simulink model "Windowlifts_2017b"  (R2017b)
settings: Solver=FixedStepDiscrete  StartTime=0.0  StopTime=inf  FixedStep=0.0001  RelTol=1e-3
model workspace (MAT data in the model file):
  BCMU_permission = Simulink.Parameter
  BCMU_permission.Value = 1
  BCMU_permission.DataType = 'boolean'
  BCMU_permission.Min = 0
  BCMU_permission.Max = 1
  BCMU_permission.Dimensions = [1 1]
  driver_win_dn = Simulink.Parameter
  driver_win_dn.Value = 0
  driver_win_dn.DataType = 'boolean'
  driver_win_dn.Dimensions = [1 1]
  driver_win_up = Simulink.Parameter
  driver_win_up.Value = 0
  driver_win_up.DataType = 'boolean'
  driver_win_up.Dimensions = [1 1]
  mir_heater = Simulink.Parameter
  mir_heater.Value = 0
  mir_heater.Description = 'Rearview mirror heater switch request'
  mir_heater.DataType = 'boolean'
  mir_heater.Dimensions = [1 1]
  pass_win_dn = Simulink.Parameter
  pass_win_dn.Value = 0
  pass_win_dn.DataType = 'boolean'
  pass_win_dn.Dimensions = [1 1]
  pass_win_up = Simulink.Parameter
  pass_win_up.Value = 0
  pass_win_up.DataType = 'boolean'
  pass_win_up.Dimensions = [1 1]
  var_0 = Simulink.Parameter
  var_0.DataType = 'auto'
  var_0.Dimensions = [0 0]
libraries: simulink x2
settings Model: Creator=macbook  LastModifiedBy=junkie

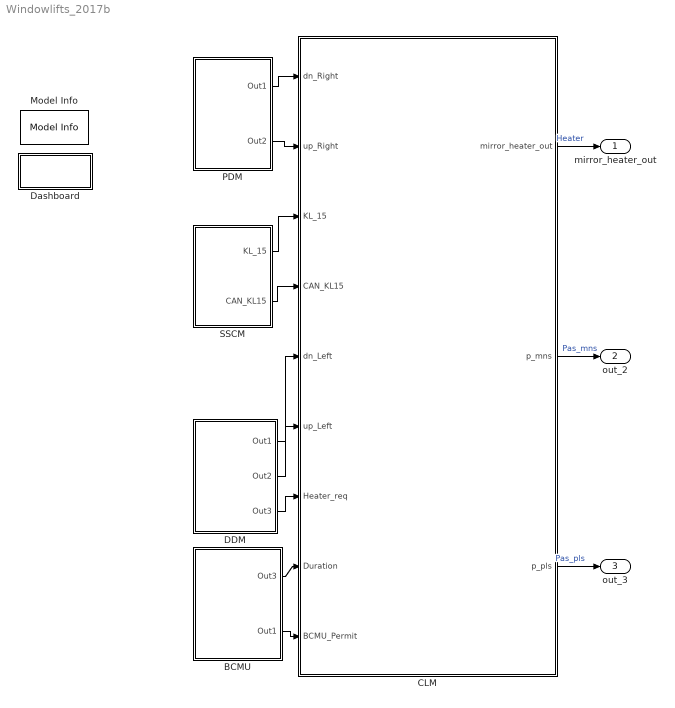
== system Windowlifts_2017b ==
  BCMU : Subsystem
  CLM : Subsystem
  DDM : Subsystem
  Dashboard : Subsystem  mask{Parameter2=<empty>}
      mask TypeOptions Parameter2: <empty>
  Model Info : simulink/Model-Wide Utilities/Model Info  Frame=on  DisplayStringWithTags=Model Info  HorizontalTextAlignment=Center  LeftAlignmentValue=0.5
  PDM : Subsystem
  SSCM : Subsystem
  mirror_heater_out : Outport
  out_2 : Outport  Port=2
  out_3 : Outport  Port=3
  wires:
  SSCM/1(KL_15) -> CLM/3(KL_15)
  SSCM/2(CAN_KL15) -> CLM/4(CAN_KL15)
  PDM/1(Out1) -> CLM/1(dn_Right)
  PDM/2(Out2) -> CLM/2(up_Right)
  DDM/1(Out1) -> CLM/5(dn_Left)
  DDM/2(Out2) -> CLM/6(up_Left)
  DDM/3(Out3) -> CLM/7(Heater_req)
  BCMU/1(Out3) -> CLM/8(Duration)
  CLM/1(mirror_heater_out) -> mirror_heater_out/1  "Heater"
  CLM/3(p_pls) -> out_3/1  "Pas_pls"
  CLM/2(p_mns) -> out_2/1  "Pas_mns"
  BCMU/2(Out1) -> CLM/9(BCMU_Permit)

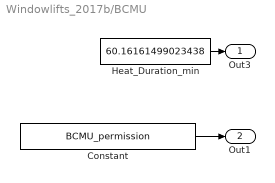
== system Windowlifts_2017b/BCMU ==
  Constant : Constant  Value=BCMU_permission
  "Heat_Duration_min " : Constant  Value=60.16161499023438  OutDataTypeStr=uint8
  Out3 : Outport
  Out1 : Outport  Port=2
  wires:
  "Heat_Duration_min "/1 -> Out3/1
  Constant/1 -> Out1/1

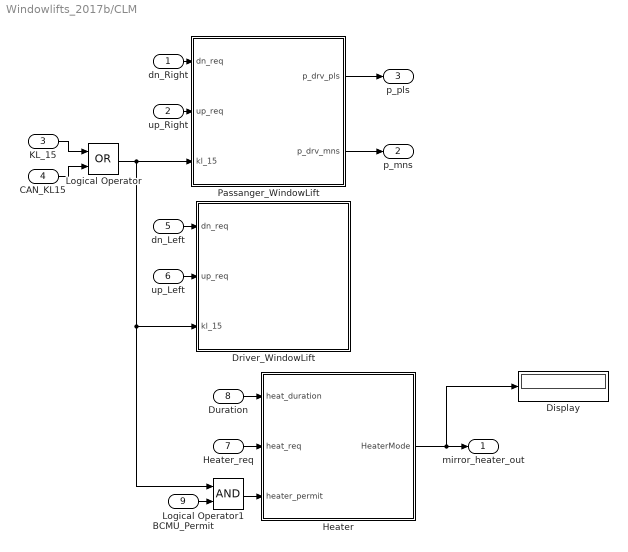
== system Windowlifts_2017b/CLM ==
  dn_Right : Inport
  up_Right : Inport  Port=2
  KL_15 : Inport  Port=3
  CAN_KL15 : Inport  Port=4
  dn_Left : Inport  Port=5
  up_Left : Inport  Port=6
  Heater_req : Inport  Port=7
  Duration : Inport  Port=8
  BCMU_Permit : Inport  Port=9
  Display : Display
  Driver_WindowLift : Stateflow chart  TreatAsAtomicUnit=on
  Heater : Stateflow chart  TreatAsAtomicUnit=on
  Logical Operator : Logic  Operator=OR  AllPortsSameDT=off  OutDataTypeStr=boolean
  Logical Operator1 : Logic  AllPortsSameDT=off  OutDataTypeStr=boolean
  Passanger_WindowLift : Stateflow chart  TreatAsAtomicUnit=on
  mirror_heater_out : Outport
  p_mns : Outport  Port=2
  p_pls : Outport  Port=3
  wires:
  dn_Right/1 -> Passanger_WindowLift/1(dn_req)
  up_Right/1 -> Passanger_WindowLift/2(up_req)
  CAN_KL15/1 -> Logical Operator/2
  up_Left/1 -> Driver_WindowLift/2(up_req)
  dn_Left/1 -> Driver_WindowLift/1(dn_req)
  KL_15/1 -> Logical Operator/1
  Heater/1(HeaterMode) -> Display/1, mirror_heater_out/1
  Duration/1 -> Heater/1(heat_duration)
  Heater_req/1 -> Heater/2(heat_req)
  Passanger_WindowLift/1(p_drv_pls) -> p_pls/1
  Passanger_WindowLift/2(p_drv_mns) -> p_mns/1
  BCMU_Permit/1 -> Logical Operator1/2
  Logical Operator/1 -> Logical Operator1/1, Driver_WindowLift/3(kl_15), Passanger_WindowLift/3(kl_15)
  Logical Operator1/1 -> Heater/3(heater_permit)

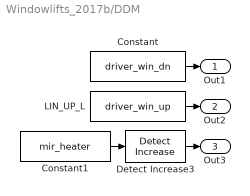
== system Windowlifts_2017b/DDM ==
  Constant : Constant  Value=driver_win_dn
  Constant1 : Constant  Value=mir_heater  OutMin=[0]  OutMax=[1]
  Detect Increase3 : simulink/Logic and Bit Operations/Detect Increase  vinit=0.0  OutDataTypeStr=boolean
  LIN_UP_L : Constant  Value=driver_win_up
  Out1 : Outport
  Out2 : Outport  Port=2
  Out3 : Outport  Port=3
  wires:
  Constant1/1 -> Detect Increase3/1
  Detect Increase3/1 -> Out3/1
  LIN_UP_L/1 -> Out2/1
  Constant/1 -> Out1/1

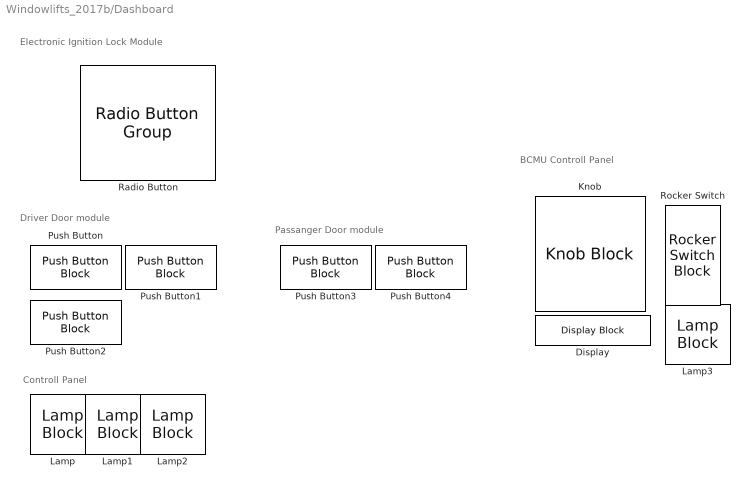
== system Windowlifts_2017b/Dashboard ==
  note: Passanger Door module
  note: Electronic Ignition Lock Module
  note: Driver Door module
  note: BCMU Controll Panel
  note: Controll Panel
  Display : DisplayBlock  WebBlockId=205  LabelPosition=Hide
  Knob : KnobBlock  WebBlockId=135  ScaleMax=120
  Lamp : LampBlock  WebBlockId=190
  Lamp1 : LampBlock  WebBlockId=191
  Lamp2 : LampBlock  WebBlockId=192
  Lamp3 : LampBlock  WebBlockId=196
  Push Button : PushButtonBlock  WebBlockId=179  ButtonText=driver_win_dn
  Push Button1 : PushButtonBlock  WebBlockId=181  ButtonText=driver_win_up
  Push Button2 : PushButtonBlock  WebBlockId=182  ButtonText=mir_heater
  Push Button3 : PushButtonBlock  WebBlockId=184  ButtonText=pass_win_dn
  Push Button4 : PushButtonBlock  WebBlockId=185  ButtonText=pass_win_up
  Radio Button : RadioButtonGroup  WebBlockId=49  SelectedLabel=IgnitionOn  ButtonGroupName=Key States
      settings: Values={{'KeyRemoved', 'KeyInserted', 'IgnitionOn'}, [0 1 2]}
  Rocker Switch : RockerSwitchBlock  WebBlockId=203
      settings: Values={{'Off', 'On'}, [0 1]}

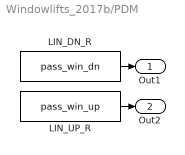
== system Windowlifts_2017b/PDM ==
  LIN_DN_R : Constant  Value=pass_win_dn
  LIN_UP_R : Constant  Value=pass_win_up
  Out1 : Outport
  Out2 : Outport  Port=2
  wires:
  LIN_UP_R/1 -> Out2/1
  LIN_DN_R/1 -> Out1/1

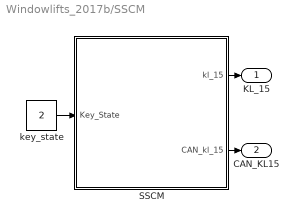
== system Windowlifts_2017b/SSCM ==
  SSCM : Stateflow chart  TreatAsAtomicUnit=on
  key_state : Constant  Value=2
  KL_15 : Outport
  CAN_KL15 : Outport  Port=2
  wires:
  SSCM/1(kl_15) -> KL_15/1
  SSCM/2(CAN_kl_15) -> CAN_KL15/1
  key_state/1 -> SSCM/1(Key_State)

== stateflow chart Windowlifts_2017b/SSCM/SSCM ==
  note: Do not put any code along
      | the transitions that run
      | down the right side!
  (default) -> (junction 74) : % StateLogic
  (junction 74) -> (junction 75) [order 1] : [Key_State ==  0]
  (junction 74) -> (junction 78) [order 2]
  (junction 75) -> (junction 76) : {kl_15 = 0;
      | CAN_kl_15 = 0}
  (junction 76) -> (junction 77)
  (junction 77) -> (junction 81)
  (junction 78) -> (junction 79) [order 1] : [Key_State == 1]
  (junction 78) -> (junction 82) [order 2]
  (junction 79) -> (junction 80) : {kl_15 = 0;
      | CAN_kl_15 = 0;}
  (junction 80) -> (junction 81)
  (junction 81) -> (junction 85)
  (junction 82) -> (junction 83) [order 1] : [Key_State ==  2]
  (junction 82) -> (junction 86) [order 2] : {kl_15 = 0;}
  (junction 83) -> (junction 84) : {kl_15 = 1;
      | CAN_kl_15 = 1}
  (junction 84) -> (junction 85)
  (junction 85) -> (junction 87)
  (junction 87) -> (junction 86)
  (junction 86) -> (junction 88)
  data: Key_State input; kl_15 output; CAN_kl_15 output

== stateflow chart Windowlifts_2017b/CLM/Driver_WindowLift ==
  note: Subsystem defines state of the system
  note: Subsystem defines the current output of the model
  note: Subsystem defines the kinematic of the drive
  state Logic [parallel]
    settings: executionOrder=1
    state up
      du:
      Current.ON;
      Kinematics.UP
    state bypass
      du:
      Current.OFF;
      Kinematics.IDLE
    state dn
      du:
      Current.ON;
      Kinematics.DN
    up -> bypass : [~up_req || dn_req || ~kl_15 ]
    bypass -> up [order 1] : [~dn_req && up_req && kl_15]
    (default) -> bypass
    dn -> bypass : [~dn_req || up_req || ~kl_15]
    bypass -> dn [order 2] : [~up_req && dn_req && kl_15]
  state Current [parallel]
    settings: executionOrder=2
    state current_on
    state current_off
    current_off -> current_on : ON
    current_on -> current_off : OFF
    (default) -> current_off
  state Kinematics [parallel]
    settings: executionOrder=3
    state idle
    state moving_down
    state moving_up
    (default) -> idle
    idle -> moving_down [order 1] : DN
    moving_down -> idle : IDLE
    idle -> moving_up [order 2] : UP
    moving_up -> idle : IDLE
  data: dn_req input; up_req input; kl_15 input
  events: ON local FUNCTION_CALL_EVENT; OFF local FUNCTION_CALL_EVENT; DN local FUNCTION_CALL_EVENT; UP local FUNCTION_CALL_EVENT; IDLE local FUNCTION_CALL_EVENT

== stateflow chart Windowlifts_2017b/CLM/Passanger_WindowLift ==
  note: Subsystem defines state of the system
  note: Subsystem defines the current output of the model
  note: Subsystem defines the kinematic of the drive
  state Logic [parallel]
    settings: executionOrder=1
    state up
      du:
      Current.ON;
      Kinematics.UP
    state bypass
      du:
      Current.OFF;
      Kinematics.IDLE
    state dn
      du:
      Current.ON;
      Kinematics.DN
    up -> bypass : [~up_req || dn_req || ~kl_15 ]
    bypass -> up [order 1] : [~dn_req && up_req && kl_15]
    (default) -> bypass
    dn -> bypass : [~dn_req || up_req || ~kl_15]
    bypass -> dn [order 2] : [~up_req && dn_req && kl_15]
  state Current [parallel]
    settings: executionOrder=2
    state current_on
    state current_off
    current_off -> current_on : ON
    current_on -> current_off : OFF
    (default) -> current_off
  state Kinematics [parallel]
    settings: executionOrder=3
    state idle
      en, du: p_drv_pls = 0;
      p_drv_mns = 0;
    state moving_down
      en, du: p_drv_pls = -1;
      p_drv_mns = 1;
    state moving_up
      en, du: p_drv_pls = 1;
      p_drv_mns = -1;
    (default) -> idle
    idle -> moving_down [order 1] : DN
    moving_down -> idle : IDLE
    idle -> moving_up [order 2] : UP
    moving_up -> idle : IDLE
  data: dn_req input; up_req input; kl_15 input; p_drv_pls output [0..1]; p_drv_mns output [0..1]
  events: ON local FUNCTION_CALL_EVENT; OFF local FUNCTION_CALL_EVENT; DN local FUNCTION_CALL_EVENT; UP local FUNCTION_CALL_EVENT; IDLE local FUNCTION_CALL_EVENT

== stateflow chart Windowlifts_2017b/CLM/Heater ==
  settings: executeAtInitialization=1
  state On_state
  state Off_state
  On_state -> Off_state [order 1] : [heat_req || ~heater_permit]
  On_state -> Off_state [order 2] : [after(heat_duration,'sec')]
  Off_state -> On_state : [heater_permit && heat_req]
  (default) -> Off_state
  data: heat_duration input; heat_req input; heater_permit input; HeaterMode output Enum: HeaterModeType
